simulink model "mslbus_28"  (Simulink 8.0)
settings: Solver=FixedStepDiscrete  StartTime=0.0  StopTime=10.0  FixedStep=0.1  RelTol=1e-3
PreLoadFcn:
  | load mslbus_28_data.mat
CloseFcn:
  | rtwprivate ssgencode ModelCloseRequest rtwssports
settings Model: FPTRunName=Active  Creator=tuschner  LastModifiedBy=qshi  ExtModeAutoUpdateStatusClock=off
settings SolverCC: AutoInsertRateTranBlk=on
settings DataIOCC: SignalLoggingSaveFormat=ModelDataLogs  SaveOutput=off  SignalLogging=off  SaveTime=off
settings OptimizationCC: InlineParams=on  InlineInvariantSignals=on  InitFltsAndDblsToZero=on  OptimizeModelRefInitCode=on  LifeSpan=1
settings DebuggingCC: SaveWithParameterizedLinksMsg=none  MultiTaskDSMMsg=warning  MultiTaskCondExecSysMsg=none  FcnCallInpInsideContextMsg=Use local settings
settings HardwareCC: TargetBitPerLong=64  TargetBitPerPointer=64  TargetEndianess=LittleEndian  TargetWordSize=64  TargetHWDeviceType=MATLAB Host  ProdEqTarget=off
settings RTWCC: SystemTargetFile=ert.tlc  TemplateMakefile=ert_default_tmf  Description=RTW Embedded Coder (no auto configuration)  RetainRTWFile=on  ProcessScript=ert_make_rtw_hook  IncludeERTFirstTime=on
settings CodeAppCC: IgnoreCustomStorageClasses=off
settings ERTTargetCC: TargetFcnLib=ansi_tfl_tmw.mat  FunctionExecutionProfile=off  MultiwordLength=2048  GenerateSampleERTMain=on  IncludeMdlTerminateFcn=off  SuppressErrorStatus=on  SupportAbsoluteTime=off  SupportNonFinite=off  SupportComplex=off  PurelyIntegerCode=on  InlinedParameterPlacement=NonHierarchical  ERTCustomFileTemplate=example_file_process.tlc  ConvertIfToSwitch=off  SupressUnreachableDefaultCases=off

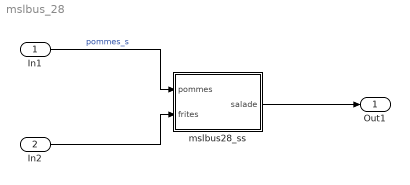
== system mslbus_28 ==
  In1 : Inport  OutDataTypeStr=pommes_t
  In2 : Inport  Port=2  OutDataTypeStr=frites_t
  mslbus28_ss : Subsystem  TreatAsAtomicUnit=on
  Out1 : Outport
  wires:
  In1/1 -> mslbus28_ss/1(pommes)  "pommes_s"
  In2/1 -> mslbus28_ss/2(frites)
  mslbus28_ss/1(salade) -> Out1/1

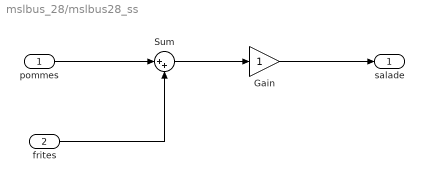
== system mslbus_28/mslbus28_ss ==
  pommes : Inport
  frites : Inport  Port=2
  Gain : Gain  OutDataTypeStr=salade_t
  Sum : Sum  Inputs=|++
  salade : Outport
  wires:
  Sum/1 -> Gain/1
  pommes/1 -> Sum/1
  Gain/1 -> salade/1
  frites/1 -> Sum/2
